simulink model "IFCC_SIMULATION"  (R2018a)
settings: Solver=VariableStepAuto  StartTime=0.0  StopTime=10.0  RelTol=1e-3
libraries: simulink x25
(part 2 of 2)

== system IFCC_SIMULATION/STATE ESTIMATION ==
  IMU PITCH : Inport
  IMU ROLL : Inport  Port=2
  IMU YAW : Inport  Port=3
  GPS ALTITUDE : Inport  Port=4
  PITOT AIRSPEED : Inport  Port=5
  AIRSPEED EKF : Subsystem
  ALTITUDE EKF : Subsystem
  PITCH EKF : Subsystem
  ROLL EKF : Subsystem
  YAW EKF : Subsystem
  ESTIMATED PITCH : Outport
  ESTIMATED ROLL : Outport  Port=2
  ESTIMATED YAW : Outport  Port=3
  ESTIMATED ALTITUDE : Outport  Port=4
  ESTIMATED AIRSPEED : Outport  Port=5
  wires:
  IMU PITCH/1 -> PITCH EKF/1(MEASURED PITCH)
  PITCH EKF/1(ESTIMATED PITCH) -> ESTIMATED PITCH/1
  GPS ALTITUDE/1 -> ALTITUDE EKF/1(MEASURED ALTITUDE)
  ROLL EKF/1(ESTIMATED ROLL) -> ESTIMATED ROLL/1
  IMU ROLL/1 -> ROLL EKF/1(MEASURED ROLL)
  IMU YAW/1 -> YAW EKF/1(MEASURED YAW)
  YAW EKF/1(ESTIMATED YAW) -> ESTIMATED YAW/1
  ALTITUDE EKF/1(ESTIMATED ALTITUDE) -> ESTIMATED ALTITUDE/1
  PITOT AIRSPEED/1 -> AIRSPEED EKF/1(MEASURED AIRSPEED)
  AIRSPEED EKF/1(ESTIMATED AIRSPEED) -> ESTIMATED AIRSPEED/1

== system IFCC_SIMULATION/AIRCRAFT PLANT/AIRSPEED DYNAMICS ==
  "THROTTLE " : Inport
  Transfer Fcn : TransferFcn  Denominator=[5 1]
  AIRSPEED : Outport
  wires:
  "THROTTLE "/1 -> Transfer Fcn/1
  Transfer Fcn/1 -> AIRSPEED/1

== system IFCC_SIMULATION/AIRCRAFT PLANT/ALTITUDE DYNAMICS ==
  PITCH : Inport
  Transfer Fcn : TransferFcn  Denominator=[10 1]
  ALTITUDE : Outport
  wires:
  PITCH/1 -> Transfer Fcn/1
  Transfer Fcn/1 -> ALTITUDE/1

== system IFCC_SIMULATION/AIRCRAFT PLANT/PITCH DYNAMICS ==
  ELEVATOR : Inport
  Transfer Fcn : TransferFcn  Denominator=[3 1]
  PITCH : Outport
  wires:
  ELEVATOR/1 -> Transfer Fcn/1
  Transfer Fcn/1 -> PITCH/1

== system IFCC_SIMULATION/AIRCRAFT PLANT/ROLL DYNAMICS ==
  AILERON : Inport
  Transfer Fcn : TransferFcn  Denominator=[2 1]
  ROLL : Outport
  wires:
  AILERON/1 -> Transfer Fcn/1
  Transfer Fcn/1 -> ROLL/1

== system IFCC_SIMULATION/AIRCRAFT PLANT/YAW DYNAMICS ==
  RUDDER : Inport
  Transfer Fcn : TransferFcn  Denominator=[4 1]
  YAW : Outport
  wires:
  RUDDER/1 -> Transfer Fcn/1
  Transfer Fcn/1 -> YAW/1

== system IFCC_SIMULATION/FLIGHT MODE MANAGER/AUTOPILOT MODES ==
  CURRENT PITCH : Inport
  MODE : Inport  Port=2
  CURRENT ALTITUDE : Inport  Port=3
  TARGET ALTITUDE : Inport  Port=4
  ALTITUDE HOLD MODE : Subsystem
  PITCH HOLD MODE : Subsystem
  PITCH HOLD OUTPUT : Outport
  ALTITUDE HOLD OUTPUT : Outport  Port=2
  wires:
  PITCH HOLD MODE/1(DESIRED PITCH) -> PITCH HOLD OUTPUT/1
  CURRENT PITCH/1 -> PITCH HOLD MODE/1(CURRENT PITCH)
  MODE/1 -> PITCH HOLD MODE/2(HOLD ENABLE)
  TARGET ALTITUDE/1 -> ALTITUDE HOLD MODE/2(TARGET ALTITUDE)
  CURRENT ALTITUDE/1 -> ALTITUDE HOLD MODE/1(CURRENT ALTITUDE)
  ALTITUDE HOLD MODE/1(DESIRED PITCH) -> ALTITUDE HOLD OUTPUT/1

== system IFCC_SIMULATION/SENSOR SIMULATION/ GPS Sensor ==
  TRUE ALTITUDE : Inport
  " Bias Adder " : Sum
  " GPS bias" : Constant  Value=0.02
  " Noise Adder" : Sum
  GPS Delay : TransportDelay  DelayTime=0.2
  GPS Noise : simulink/Sources/Band-Limited White Noise  Cov=1e-5  Ts=0.1  seed=45678
  GPS ALTITUDE : Outport
  wires:
  TRUE ALTITUDE/1 -> GPS Delay/1
  GPS Noise/1 -> " Noise Adder"/1
  GPS Delay/1 -> " Noise Adder"/2
  " Noise Adder"/1 -> " Bias Adder "/1
  " GPS bias"/1 -> " Bias Adder "/2
  " Bias Adder "/1 -> GPS ALTITUDE/1

== system IFCC_SIMULATION/SENSOR SIMULATION/ IMU Pitch Sensor  ==
  TRUE ANGLE : Inport
  " Bias Adder" : Sum
  " Noise Adder" : Sum
  " Bias" : Constant  Value=0.005
  Measurement Noise : simulink/Sources/Band-Limited White Noise  Cov=1e-6  Ts=0.01  seed=12345
  MEASURED ANGLE : Outport
  wires:
  " Bias Adder"/1 -> MEASURED ANGLE/1
  Measurement Noise/1 -> " Noise Adder"/1
  " Noise Adder"/1 -> " Bias Adder"/2
  " Bias"/1 -> " Bias Adder"/1
  TRUE ANGLE/1 -> " Noise Adder"/2

== system IFCC_SIMULATION/SENSOR SIMULATION/ IMU Roll Sensor ==
  TRUE ANGLE : Inport
  " Pitch Bias Adder" : Sum
  " Pitch Noise Adder" : Sum
  Pitch Noise : simulink/Sources/Band-Limited White Noise  Cov=1e-6  Ts=0.01  seed=23456
  Pitch bias : Constant  Value=0.005
  MEASURED ANGLE : Outport
  wires:
  " Pitch Bias Adder"/1 -> MEASURED ANGLE/1
  Pitch Noise/1 -> " Pitch Noise Adder"/1
  " Pitch Noise Adder"/1 -> " Pitch Bias Adder"/2
  Pitch bias/1 -> " Pitch Bias Adder"/1
  TRUE ANGLE/1 -> " Pitch Noise Adder"/2

== system IFCC_SIMULATION/SENSOR SIMULATION/ IMU Yaw Sensor ==
  TRUE ANGLE : Inport
  " Pitch Bias Adder" : Sum
  " Pitch Noise Adder" : Sum
  Pitch Noise : simulink/Sources/Band-Limited White Noise  Cov=1e-6  Ts=0.01  seed=34567
  Pitch bias : Constant  Value=0.005
  MEASURED ANGLE : Outport
  wires:
  " Pitch Bias Adder"/1 -> MEASURED ANGLE/1
  Pitch Noise/1 -> " Pitch Noise Adder"/1
  " Pitch Noise Adder"/1 -> " Pitch Bias Adder"/2
  Pitch bias/1 -> " Pitch Bias Adder"/1
  TRUE ANGLE/1 -> " Pitch Noise Adder"/2

== system IFCC_SIMULATION/SENSOR SIMULATION/PITOT AIRSPEED SENSOR ==
  TRUE AIRSPEED : Inport
  " Bias Adder" : Sum
  " Noise Adder" : Sum
  " Bias" : Constant  Value=0.02
  Measurement Noise : simulink/Sources/Band-Limited White Noise  Cov=1e-6  Ts=0.01  seed=12345
  PITOT AIRSPEED : Outport
  wires:
  " Noise Adder"/1 -> " Bias Adder"/2
  TRUE AIRSPEED/1 -> " Noise Adder"/2
  " Bias"/1 -> " Bias Adder"/1
  " Bias Adder"/1 -> PITOT AIRSPEED/1
  Measurement Noise/1 -> " Noise Adder"/1

== system IFCC_SIMULATION/STATE ESTIMATION/AIRSPEED EKF ==
  MEASURED AIRSPEED : Inport
  CORRECTION STEP : Subsystem
  COVARIANCE MEMORY : UnitDelay  InitialCondition=1  SampleTime=-1
  MEASUREMENT NOISE(R) : Constant  Value=0.01
  PREDICTION STEP : Subsystem
  STATE MEMORY : UnitDelay  SampleTime=-1
  ESTIMATED AIRSPEED : Outport
  wires:
  MEASURED AIRSPEED/1 -> CORRECTION STEP/3(MEASURED AIRSPEED)
  STATE MEMORY/1 -> PREDICTION STEP/1(PREVIOUS STATE)
  PREDICTION STEP/2(PREDICTED COVARIANCE) -> CORRECTION STEP/2(PREDICTED COVARIANCE)
  COVARIANCE MEMORY/1 -> PREDICTION STEP/2(PREVIOUS COVARIANCE)
  CORRECTION STEP/2(UPDATED COVARIANCE) -> COVARIANCE MEMORY/1
  PREDICTION STEP/1(PREDICTED STATE) -> CORRECTION STEP/1(PREDICTED STATE)
  MEASUREMENT NOISE(R)/1 -> CORRECTION STEP/4(MEASUREMENT COVARIANCE)
  CORRECTION STEP/1(UPDATED STATE) -> ESTIMATED AIRSPEED/1, STATE MEMORY/1

== system IFCC_SIMULATION/STATE ESTIMATION/ALTITUDE EKF ==
  MEASURED ALTITUDE : Inport
  CORRECTION STEP : Subsystem
  COVARIANCE MEMORY : UnitDelay  InitialCondition=1  SampleTime=-1
  MEASUREMENT NOISE(R) : Constant  Value=0.01
  PREDICTION STEP : Subsystem
  STATE MEMORY : UnitDelay  SampleTime=-1
  ESTIMATED ALTITUDE : Outport
  wires:
  MEASURED ALTITUDE/1 -> CORRECTION STEP/3(MEASURED ALTITUDE)
  STATE MEMORY/1 -> PREDICTION STEP/1(PREVIOUS STATE)
  PREDICTION STEP/2(PREDICTED COVARIANCE) -> CORRECTION STEP/2(PREDICTED COVARIANCE)
  COVARIANCE MEMORY/1 -> PREDICTION STEP/2(PREVIOUS COVARIANCE)
  CORRECTION STEP/2(UPDATED COVARIANCE) -> COVARIANCE MEMORY/1
  PREDICTION STEP/1(PREDICTED STATE) -> CORRECTION STEP/1(PREDICTED STATE)
  MEASUREMENT NOISE(R)/1 -> CORRECTION STEP/4(MEASUREMENT COVARIANCE)
  CORRECTION STEP/1(UPDATED STATE) -> ESTIMATED ALTITUDE/1, STATE MEMORY/1

== system IFCC_SIMULATION/STATE ESTIMATION/PITCH EKF ==
  MEASURED PITCH : Inport
  CORRECTION STEP : Subsystem
  COVARIANCE MEMORY : UnitDelay  InitialCondition=1  SampleTime=-1
  MEASUREMENT NOISE(R) : Constant  Value=0.01
  PREDICTION STEP : Subsystem
  STATE MEMORY : UnitDelay  SampleTime=-1
  ESTIMATED PITCH : Outport
  wires:
  STATE MEMORY/1 -> PREDICTION STEP/1(PREVIOUS STATE)
  COVARIANCE MEMORY/1 -> PREDICTION STEP/2(PREVIOUS COVARIANCE)
  CORRECTION STEP/2(UPDATED COVARIANCE) -> COVARIANCE MEMORY/1
  MEASUREMENT NOISE(R)/1 -> CORRECTION STEP/4(MEASUREMENT COVARIANCE)
  PREDICTION STEP/1(PREDICTED STATE) -> CORRECTION STEP/1(PREDICTED STATE)
  PREDICTION STEP/2(PREDICTED COVARIANCE) -> CORRECTION STEP/2(PREDICTED COVARIANCE)
  MEASURED PITCH/1 -> CORRECTION STEP/3(MEASURED PITCH)
  CORRECTION STEP/1(UPDATED STATE) -> ESTIMATED PITCH/1, STATE MEMORY/1

== system IFCC_SIMULATION/STATE ESTIMATION/ROLL EKF ==
  MEASURED ROLL : Inport
  CORRECTION STEP : Subsystem
  COVARIANCE MEMORY : UnitDelay  InitialCondition=1  SampleTime=-1
  MEASUREMENT NOISE(R) : Constant  Value=0.01
  PREDICTION STEP : Subsystem
  STATE MEMORY : UnitDelay  SampleTime=-1
  ESTIMATED ROLL : Outport
  wires:
  PREDICTION STEP/2(PREDICTED COVARIANCE) -> CORRECTION STEP/2(PREDICTED COVARIANCE)
  COVARIANCE MEMORY/1 -> PREDICTION STEP/2(PREVIOUS COVARIANCE)
  CORRECTION STEP/2(UPDATED COVARIANCE) -> COVARIANCE MEMORY/1
  PREDICTION STEP/1(PREDICTED STATE) -> CORRECTION STEP/1(PREDICTED STATE)
  STATE MEMORY/1 -> PREDICTION STEP/1(PREVIOUS STATE)
  MEASURED ROLL/1 -> CORRECTION STEP/3(MEASURED ROLL)
  CORRECTION STEP/1(UPDATED STATE) -> ESTIMATED ROLL/1, STATE MEMORY/1
  MEASUREMENT NOISE(R)/1 -> CORRECTION STEP/4(MEASUREMENT COVARIANCE)

== system IFCC_SIMULATION/STATE ESTIMATION/YAW EKF ==
  MEASURED YAW : Inport
  CORRECTION STEP : Subsystem
  COVARIANCE MEMORY : UnitDelay  InitialCondition=1  SampleTime=-1
  MEASUREMENT NOISE(R) : Constant  Value=0.01
  PREDICTION STEP : Subsystem
  STATE MEMORY : UnitDelay  SampleTime=-1
  ESTIMATED YAW : Outport
  wires:
  PREDICTION STEP/2(PREDICTED COVARIANCE) -> CORRECTION STEP/2(PREDICTED COVARIANCE)
  COVARIANCE MEMORY/1 -> PREDICTION STEP/2(PREVIOUS COVARIANCE)
  CORRECTION STEP/2(UPDATED COVARIANCE) -> COVARIANCE MEMORY/1
  PREDICTION STEP/1(PREDICTED STATE) -> CORRECTION STEP/1(PREDICTED STATE)
  STATE MEMORY/1 -> PREDICTION STEP/1(PREVIOUS STATE)
  MEASURED YAW/1 -> CORRECTION STEP/3(MEASURED YAW)
  CORRECTION STEP/1(UPDATED STATE) -> ESTIMATED YAW/1, STATE MEMORY/1
  MEASUREMENT NOISE(R)/1 -> CORRECTION STEP/4(MEASUREMENT COVARIANCE)

== system IFCC_SIMULATION/FLIGHT MODE MANAGER/AUTOPILOT MODES/ALTITUDE HOLD MODE ==
  CURRENT ALTITUDE : Inport
  TARGET ALTITUDE : Inport  Port=2
  " ALTITUDE ERROR" : Sum  Inputs=+-
  ALTITUDE PID : simulink/Continuous/PID Controller  Controller=PID  TimeDomain=Continuous-time  SampleTime=-1  IntegratorMethod=Forward Euler  FilterMethod=Forward Euler  Form=Parallel  UseFilter=on  ControllerParametersSource=internal  P=1  I=1  D=0  N=100  InitialConditionSource=internal  InitialConditionForIntegrator=0  InitialConditionForFilter=0  ExternalReset=none  LimitOutput=off  UpperSaturationLimit=inf  LowerSaturationLimit=-inf  LinearizeAsGain=on  AntiWindupMode=none  Kb=1  TrackingMode=off  Kt=1  PParamMin=[]  PParamMax=[]  IParamMin=[]  IParamMax=[]  DParamMin=[]  DParamMax=[]  NParamMin=[]  NParamMax=[]  KbParamMin=[]  KbParamMax=[]  KtParamMin=[]  KtParamMax=[]  POutMin=[]  POutMax=[]  IOutMin=[]  IOutMax=[]  DOutMin=[]  DOutMax=[]  NOutMin=[]  NOutMax=[]  KbOutMin=[]  KbOutMax=[]  KtOutMin=[]  KtOutMax=[]  IntegratorOutMin=[]  IntegratorOutMax=[]  FilterOutMin=[]  FilterOutMax=[]  SumOutMin=[]  SumOutMax=[]  SumI1OutMin=[]  SumI1OutMax=[]  SumI2OutMin=[]  SumI2OutMax=[]  SumI3OutMin=[]  SumI3OutMax=[]  SumDOutMin=[]  SumDOutMax=[]  SaturationOutMin=[]  SaturationOutMax=[]  IntegratorContinuousStateAttributes=''  IntegratorStateMustResolveToSignalObject=off  IntegratorRTWStateStorageClass=Auto  FilterContinuousStateAttributes=''  FilterStateMustResolveToSignalObject=off  FilterRTWStateStorageClass=Auto  DifferentiatorICPrevScaledInput=0  DifferentiatorOutMin=[]  DifferentiatorOutMax=[]  FilterDiffOutCoefMin=[]  FilterDiffOutCoefMax=[]  SumDenOutMin=[]  SumDenOutMax=[]  SumNumOutMin=[]  SumNumOutMax=[]  ReciprocalOutMin=[]  ReciprocalOutMax=[]  DivideOutMin=[]  DivideOutMax=[]  TunerSelectOption=Transfer Function Based (PID Tuner App)
  PITCH LIMIT : Saturate  UpperLimit=15  LowerLimit=-15
  DESIRED PITCH : Outport
  wires:
  TARGET ALTITUDE/1 -> " ALTITUDE ERROR"/1
  CURRENT ALTITUDE/1 -> " ALTITUDE ERROR"/2
  ALTITUDE PID/1 -> PITCH LIMIT/1
  PITCH LIMIT/1 -> DESIRED PITCH/1
  " ALTITUDE ERROR"/1 -> ALTITUDE PID/1

== system IFCC_SIMULATION/FLIGHT MODE MANAGER/AUTOPILOT MODES/PITCH HOLD MODE ==
  CURRENT PITCH : Inport
  HOLD ENABLE : Inport  Port=2
  HOLD SWITCH : Switch  Criteria=u2 > Threshold  Threshold=0.5
  PITCH MEMORY : UnitDelay  SampleTime=-1
  DESIRED PITCH : Outport
  wires:
  CURRENT PITCH/1 -> HOLD SWITCH/1
  HOLD ENABLE/1 -> HOLD SWITCH/2
  PITCH MEMORY/1 -> HOLD SWITCH/3
  HOLD SWITCH/1 -> PITCH MEMORY/1, DESIRED PITCH/1

== system IFCC_SIMULATION/STATE ESTIMATION/AIRSPEED EKF/CORRECTION STEP ==
  PREDICTED STATE : Inport
  PREDICTED COVARIANCE : Inport  Port=2
  MEASURED AIRSPEED : Inport  Port=3
  MEASUREMENT COVARIANCE : Inport  Port=4
  EKF MEASUREMENT UPDATE : MATLAB Function  TreatAsAtomicUnit=on
  UPDATED STATE : Outport
  UPDATED COVARIANCE : Outport  Port=2
  wires:
  PREDICTED STATE/1 -> EKF MEASUREMENT UPDATE/1(predicted_state)
  PREDICTED COVARIANCE/1 -> EKF MEASUREMENT UPDATE/2(predicted_covariance)
  MEASURED AIRSPEED/1 -> EKF MEASUREMENT UPDATE/3(measured_values)
  MEASUREMENT COVARIANCE/1 -> EKF MEASUREMENT UPDATE/4(R)
  EKF MEASUREMENT UPDATE/1(updated_state) -> UPDATED STATE/1
  EKF MEASUREMENT UPDATE/2(updated_covariance) -> UPDATED COVARIANCE/1

== system IFCC_SIMULATION/STATE ESTIMATION/AIRSPEED EKF/PREDICTION STEP ==
  PREVIOUS STATE : Inport
  PREVIOUS COVARIANCE : Inport  Port=2
  A : Gain
  ADD Q : Sum
  AT : Gain
  PROCESS NOISE : Constant  Value=0.001
  STATE TRANSITION : Gain
  PREDICTED STATE : Outport
  PREDICTED COVARIANCE : Outport  Port=2
  wires:
  PREVIOUS STATE/1 -> STATE TRANSITION/1
  STATE TRANSITION/1 -> PREDICTED STATE/1
  PREVIOUS COVARIANCE/1 -> A/1
  A/1 -> AT/1
  AT/1 -> ADD Q/1
  PROCESS NOISE/1 -> ADD Q/2
  ADD Q/1 -> PREDICTED COVARIANCE/1

== system IFCC_SIMULATION/STATE ESTIMATION/ALTITUDE EKF/CORRECTION STEP ==
  PREDICTED STATE : Inport
  PREDICTED COVARIANCE : Inport  Port=2
  MEASURED ALTITUDE : Inport  Port=3
  MEASUREMENT COVARIANCE : Inport  Port=4
  EKF MEASUREMENT UPDATE : MATLAB Function  TreatAsAtomicUnit=on
  UPDATED STATE : Outport
  UPDATED COVARIANCE : Outport  Port=2
  wires:
  PREDICTED STATE/1 -> EKF MEASUREMENT UPDATE/1(predicted_state)
  PREDICTED COVARIANCE/1 -> EKF MEASUREMENT UPDATE/2(predicted_covariance)
  MEASURED ALTITUDE/1 -> EKF MEASUREMENT UPDATE/3(measured_values)
  MEASUREMENT COVARIANCE/1 -> EKF MEASUREMENT UPDATE/4(R)
  EKF MEASUREMENT UPDATE/1(updated_state) -> UPDATED STATE/1
  EKF MEASUREMENT UPDATE/2(updated_covariance) -> UPDATED COVARIANCE/1

== system IFCC_SIMULATION/STATE ESTIMATION/ALTITUDE EKF/PREDICTION STEP ==
  PREVIOUS STATE : Inport
  PREVIOUS COVARIANCE : Inport  Port=2
  A : Gain
  ADD Q : Sum
  AT : Gain
  PROCESS NOISE : Constant  Value=0.001
  STATE TRANSITION : Gain
  PREDICTED STATE : Outport
  PREDICTED COVARIANCE : Outport  Port=2
  wires:
  PREVIOUS STATE/1 -> STATE TRANSITION/1
  STATE TRANSITION/1 -> PREDICTED STATE/1
  PREVIOUS COVARIANCE/1 -> A/1
  A/1 -> AT/1
  AT/1 -> ADD Q/1
  PROCESS NOISE/1 -> ADD Q/2
  ADD Q/1 -> PREDICTED COVARIANCE/1

== system IFCC_SIMULATION/STATE ESTIMATION/PITCH EKF/CORRECTION STEP ==
  PREDICTED STATE : Inport
  PREDICTED COVARIANCE : Inport  Port=2
  MEASURED PITCH : Inport  Port=3
  MEASUREMENT COVARIANCE : Inport  Port=4
  EKF MEASUREMENT UPDATE : MATLAB Function  TreatAsAtomicUnit=on
  UPDATED STATE : Outport
  UPDATED COVARIANCE : Outport  Port=2
  wires:
  PREDICTED STATE/1 -> EKF MEASUREMENT UPDATE/1(predicted_state)
  PREDICTED COVARIANCE/1 -> EKF MEASUREMENT UPDATE/2(predicted_covariance)
  MEASURED PITCH/1 -> EKF MEASUREMENT UPDATE/3(measured_pitch)
  MEASUREMENT COVARIANCE/1 -> EKF MEASUREMENT UPDATE/4(R)
  EKF MEASUREMENT UPDATE/1(updated_state) -> UPDATED STATE/1
  EKF MEASUREMENT UPDATE/2(updated_covariance) -> UPDATED COVARIANCE/1

== system IFCC_SIMULATION/STATE ESTIMATION/PITCH EKF/PREDICTION STEP ==
  PREVIOUS STATE : Inport
  PREVIOUS COVARIANCE : Inport  Port=2
  A : Gain
  ADD Q : Sum
  AT : Gain
  PROCESS NOISE : Constant  Value=0.001
  STATE TRANSITION : Gain
  PREDICTED STATE : Outport
  PREDICTED COVARIANCE : Outport  Port=2
  wires:
  PREVIOUS STATE/1 -> STATE TRANSITION/1
  STATE TRANSITION/1 -> PREDICTED STATE/1
  PREVIOUS COVARIANCE/1 -> A/1
  A/1 -> AT/1
  AT/1 -> ADD Q/1
  PROCESS NOISE/1 -> ADD Q/2
  ADD Q/1 -> PREDICTED COVARIANCE/1

== system IFCC_SIMULATION/STATE ESTIMATION/ROLL EKF/CORRECTION STEP ==
  PREDICTED STATE : Inport
  PREDICTED COVARIANCE : Inport  Port=2
  MEASURED ROLL : Inport  Port=3
  MEASUREMENT COVARIANCE : Inport  Port=4
  EKF MEASUREMENT UPDATE : MATLAB Function  TreatAsAtomicUnit=on
  UPDATED STATE : Outport
  UPDATED COVARIANCE : Outport  Port=2
  wires:
  PREDICTED STATE/1 -> EKF MEASUREMENT UPDATE/1(predicted_state)
  PREDICTED COVARIANCE/1 -> EKF MEASUREMENT UPDATE/2(predicted_covariance)
  MEASURED ROLL/1 -> EKF MEASUREMENT UPDATE/3(measured_values)
  MEASUREMENT COVARIANCE/1 -> EKF MEASUREMENT UPDATE/4(R)
  EKF MEASUREMENT UPDATE/1(updated_state) -> UPDATED STATE/1
  EKF MEASUREMENT UPDATE/2(updated_covariance) -> UPDATED COVARIANCE/1

== system IFCC_SIMULATION/STATE ESTIMATION/ROLL EKF/PREDICTION STEP ==
  PREVIOUS STATE : Inport
  PREVIOUS COVARIANCE : Inport  Port=2
  A : Gain
  ADD Q : Sum
  AT : Gain
  PROCESS NOISE : Constant  Value=0.001
  STATE TRANSITION : Gain
  PREDICTED STATE : Outport
  PREDICTED COVARIANCE : Outport  Port=2
  wires:
  PREVIOUS STATE/1 -> STATE TRANSITION/1
  STATE TRANSITION/1 -> PREDICTED STATE/1
  PREVIOUS COVARIANCE/1 -> A/1
  A/1 -> AT/1
  AT/1 -> ADD Q/1
  PROCESS NOISE/1 -> ADD Q/2
  ADD Q/1 -> PREDICTED COVARIANCE/1

== system IFCC_SIMULATION/STATE ESTIMATION/YAW EKF/CORRECTION STEP ==
  PREDICTED STATE : Inport
  PREDICTED COVARIANCE : Inport  Port=2
  MEASURED YAW : Inport  Port=3
  MEASUREMENT COVARIANCE : Inport  Port=4
  EKF MEASUREMENT UPDATE : MATLAB Function  TreatAsAtomicUnit=on
  UPDATED STATE : Outport
  UPDATED COVARIANCE : Outport  Port=2
  wires:
  PREDICTED STATE/1 -> EKF MEASUREMENT UPDATE/1(predicted_state)
  PREDICTED COVARIANCE/1 -> EKF MEASUREMENT UPDATE/2(predicted_covariance)
  MEASURED YAW/1 -> EKF MEASUREMENT UPDATE/3(measured_values)
  MEASUREMENT COVARIANCE/1 -> EKF MEASUREMENT UPDATE/4(R)
  EKF MEASUREMENT UPDATE/1(updated_state) -> UPDATED STATE/1
  EKF MEASUREMENT UPDATE/2(updated_covariance) -> UPDATED COVARIANCE/1

== system IFCC_SIMULATION/STATE ESTIMATION/YAW EKF/PREDICTION STEP ==
  PREVIOUS STATE : Inport
  PREVIOUS COVARIANCE : Inport  Port=2
  A : Gain
  ADD Q : Sum
  AT : Gain
  PROCESS NOISE : Constant  Value=0.001
  STATE TRANSITION : Gain
  PREDICTED STATE : Outport
  PREDICTED COVARIANCE : Outport  Port=2
  wires:
  PREVIOUS STATE/1 -> STATE TRANSITION/1
  STATE TRANSITION/1 -> PREDICTED STATE/1
  PREVIOUS COVARIANCE/1 -> A/1
  A/1 -> AT/1
  AT/1 -> ADD Q/1
  PROCESS NOISE/1 -> ADD Q/2
  ADD Q/1 -> PREDICTED COVARIANCE/1

== matlab function IFCC_SIMULATION/STATE ESTIMATION/ROLL EKF/CORRECTION STEP/EKF MEASUREMENT UPDATE ==
  data: predicted_state input; updated_state output; predicted_covariance input; measured_values input; R input; updated_covariance output
function [updated_state,updated_covariance] = ...
KF_Update(predicted_state,predicted_covariance,measured_values,R)

innovation = measured_values - predicted_state;

S = predicted_covariance + R;

K = predicted_covariance / S;

updated_state = predicted_state + K*innovation;

updated_covariance = (1-K)*predicted_covariance;

== matlab function IFCC_SIMULATION/STATE ESTIMATION/PITCH EKF/CORRECTION STEP/EKF MEASUREMENT UPDATE ==
  data: predicted_state input; updated_state output; predicted_covariance input; measured_pitch input; R input; updated_covariance output
function [updated_state,updated_covariance] = ...
KF_Update(predicted_state,predicted_covariance,measured_pitch,R)

innovation = measured_pitch - predicted_state;

S = predicted_covariance + R;

K = predicted_covariance / S;

updated_state = predicted_state + K*innovation;

updated_covariance = (1-K)*predicted_covariance;

== matlab function IFCC_SIMULATION/STATE ESTIMATION/YAW EKF/CORRECTION STEP/EKF MEASUREMENT UPDATE ==
  data: predicted_state input; updated_state output; predicted_covariance input; measured_values input; R input; updated_covariance output
function [updated_state,updated_covariance] = ...
KF_Update(predicted_state,predicted_covariance,measured_values,R)

innovation = measured_values - predicted_state;

S = predicted_covariance + R;

K = predicted_covariance / S;

updated_state = predicted_state + K*innovation;

updated_covariance = (1-K)*predicted_covariance;

== matlab function IFCC_SIMULATION/STATE ESTIMATION/ALTITUDE EKF/CORRECTION STEP/EKF MEASUREMENT UPDATE ==
  data: predicted_state input; updated_state output; predicted_covariance input; measured_values input; R input; updated_covariance output
function [updated_state,updated_covariance] = ...
KF_Update(predicted_state,predicted_covariance,measured_values,R)

innovation = measured_values - predicted_state;

S = predicted_covariance + R;

K = predicted_covariance / S;

updated_state = predicted_state + K*innovation;

updated_covariance = (1-K)*predicted_covariance;

== matlab function IFCC_SIMULATION/STATE ESTIMATION/AIRSPEED EKF/CORRECTION STEP/EKF MEASUREMENT UPDATE ==
  data: predicted_state input; updated_state output; predicted_covariance input; measured_values input; R input; updated_covariance output
function [updated_state,updated_covariance] = ...
KF_Update(predicted_state,predicted_covariance,measured_values,R)

innovation = measured_values - predicted_state;

S = predicted_covariance + R;

K = predicted_covariance / S;

updated_state = predicted_state + K*innovation;

updated_covariance = (1-K)*predicted_covariance;
